simulink model "Stateflow_Mealy_example"  (R2014a)
settings: Solver=FixedStepDiscrete  StartTime=0.0  StopTime=10.0  RelTol=1e-3
settings Model: Creator=mprior  LastModifiedBy=mprior
settings DataIOCC: LimitDataPoints=off  SaveOutput=off  SaveTime=off
settings DebuggingCC: SolverPrmCheckMsg=none  SingleTaskRateTransMsg=error

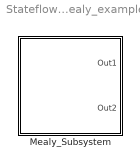
== system Stateflow_Mealy_example ==
  Mealy_Subsystem : Subsystem

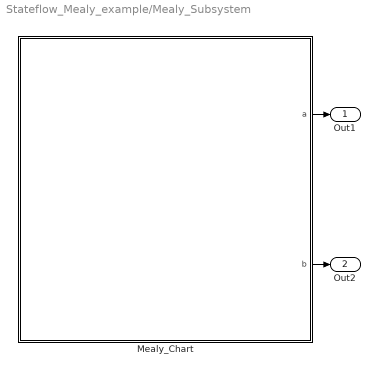
== system Stateflow_Mealy_example/Mealy_Subsystem ==
  Mealy_Chart : Stateflow chart  TreatAsAtomicUnit=on
  Out1 : Outport
  Out2 : Outport  Port=2
  wires:
  Mealy_Chart/2(b) -> Out2/1
  Mealy_Chart/1(a) -> Out1/1

== stateflow chart Stateflow_Mealy_example/Mealy_Subsystem/Mealy_Chart ==
  settings: stateMachineType=MEALY_MACHINE  executeAtInitialization=1
  state INITIAL
  state IDLE
  state FINAL
  state SEQ1
  state SEQ2
  (default) -> INITIAL
  INITIAL -> IDLE : {a=0; b=0}
  FINAL -> IDLE
  IDLE -> SEQ1 : {a=0;}
  SEQ2 -> FINAL
  SEQ1 -> SEQ2 : {a=1; b=b+1}
  data: a output double; b output double
